simulink model "PRACTICA 1"  (R2024a)
settings: Solver=ode23  StartTime=0.0  StopTime=200  RelTol=1e-3
values from neighbouring files (symbols this model uses):
  g = 9.81    [CONDICIONES.m]
  l1 = 0.3    [CONDICIONES.m]
  l2 = 0.25    [CONDICIONES.m]
  m1 = 0.2    [CONDICIONES.m]
  m2 = 0.1    [CONDICIONES.m]
settings Model: Creator=Charles  LastModifiedBy=JUAN CARLOS
settings SolverCC: AlgebraicLoopSolver=TrustRegion
settings DataIOCC: ReturnWorkspaceOutputs=off
settings DebuggingCC: UnconnectedInputMsg=warning  UnconnectedOutputMsg=warning  UnconnectedLineMsg=warning  ArithmeticOperatorsInVariantConditions=warning
settings ModelReferenceCC: EnableRefExpFcnMdlSchedulingChecks=on
settings SFSimCC: SimUseLocalCustomCode=off  CustomCodeUndefinedFunction=UseInterfaceOnly
settings RTWCC: RTWUseLocalCustomCode=off  GPUComputeCapability=3.5

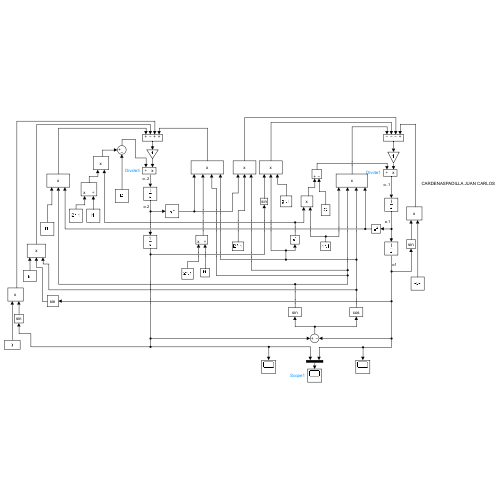
[thumbnail: Simulink's stored preview of the top-level diagram]
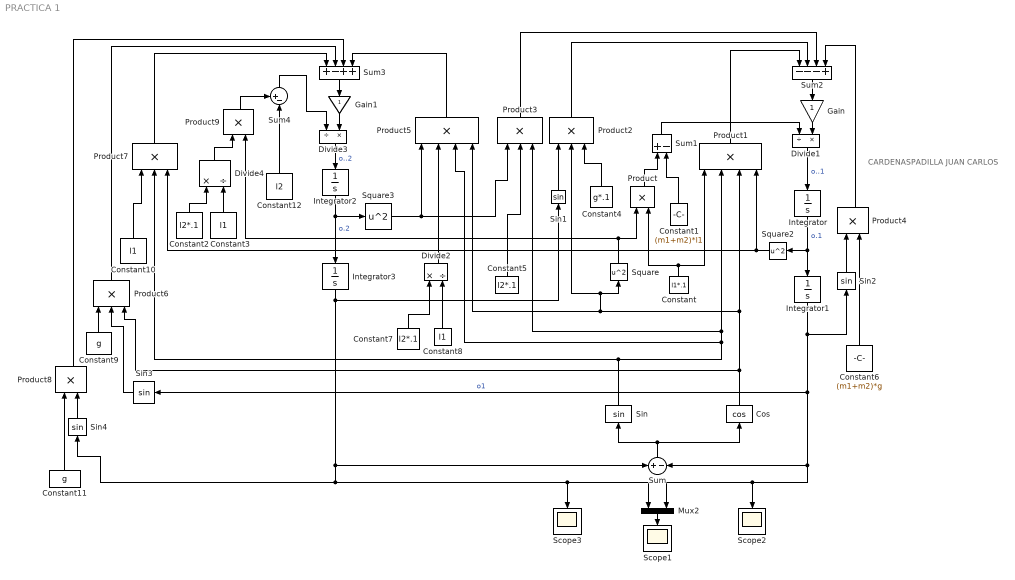
== system PRACTICA 1 ==
  note: CARDENASPADILLA JUAN CARLOS
  Constant : Constant  Value=l1*.1
  Constant1 : Constant  Value=(m1+m2)*l1
  Constant10 : Constant  Value=l1
  Constant11 : Constant  Value=g
  Constant12 : Constant  Value=l2
  Constant2 : Constant  Value=l2*.1
  Constant3 : Constant  Value=l1
  Constant4 : Constant  Value=g*.1
  Constant5 : Constant  Value=l2*.1
  Constant6 : Constant  Value=(m1+m2)*g
  Constant7 : Constant  Value=l2*.1
  Constant8 : Constant  Value=l1
  Constant9 : Constant  Value=g
  Cos : Trigonometry  Operator=cos
  Divide1 : Product  Inputs=/*
  Divide2 : Product  Inputs=*/
  Divide3 : Product  Inputs=/*
  Divide4 : Product  Inputs=*/
  Gain : Gain
  Gain1 : Gain
  Integrator : Integrator
  Integrator1 : Integrator
  Integrator2 : Integrator
  Integrator3 : Integrator  InitialCondition=0.610865
  Mux2 : Mux  Inputs=2
  Product{,4,8..9} (4 alike) : Product
  Product1 : Product  Inputs=4
  Product{2..3,6..7} (4 alike) : Product  Inputs=3
  Product5 : Product  Inputs=4
  Scope1 : Scope
  Scope2 : Scope
  Scope3 : Scope
  Sin{,1..4} (5 alike) : Trigonometry
  Square : Math  Operator=square  SignedPower=on  RndMeth=Zero
  Square2 : Math  Operator=square  SignedPower=on  RndMeth=Zero
  Square3 : Math  Operator=square  SignedPower=on  RndMeth=Zero
  Sum : Sum  Inputs=+-
  Sum1 : Sum  Inputs=+-
  Sum2 : Sum  Inputs=---+
  Sum3 : Sum  Inputs=+-++
  Sum4 : Sum  Inputs=+-|
  wires:
  Gain/1 -> Divide1/2
  Integrator/1 -> Integrator1/1, Square2/1  "o.1"
  Integrator1/1 -> Scope2/1, Mux2/2, Sum/2, Sin3/1, Sin2/1  "o1"
  Integrator2/1 -> Integrator3/1, Square3/1  "o.2"
  Integrator3/1 -> Sin4/1, Mux2/1, Scope3/1, Sum/1, Sin1/1
  Gain1/1 -> Divide3/2
  Sum/1 -> Cos/1, Sin/1
  Cos/1 -> Product6/3, Product2/2, Square/1, Product5/4, Product1/3
  Sin/1 -> Product5/3, Product3/3, Product1/2, Product7/2
  Square/1 -> Product/1, Product9/2
  Constant/1 -> Product1/1, Product/2
  Constant1/1 -> Sum1/2
  Product/1 -> Sum1/1
  Sum1/1 -> Divide1/1
  Divide1/1 -> Integrator/1  "o..1"
  Square2/1 -> Product1/4, Product7/3
  Product1/1 -> Sum2/1
  Sin1/1 -> Product2/1
  Constant4/1 -> Product2/3
  Product2/1 -> Sum2/2
  Constant5/1 -> Product3/2
  Square3/1 -> Product5/1, Product3/1
  Product3/1 -> Sum2/3
  Sin2/1 -> Product4/1
  Constant6/1 -> Product4/2
  Product4/1 -> Sum2/4
  Sum3/1 -> Gain1/1
  Constant8/1 -> Divide2/2
  Constant7/1 -> Divide2/1
  Divide2/1 -> Product5/2
  Product5/1 -> Sum3/4
  Sin3/1 -> Product6/2
  Constant9/1 -> Product6/1
  Constant10/1 -> Product7/1
  Product7/1 -> Sum3/1
  Product6/1 -> Sum3/2
  Sin4/1 -> Product8/2
  Constant11/1 -> Product8/1
  Product8/1 -> Sum3/3
  Divide3/1 -> Integrator2/1  "o..2"
  Constant2/1 -> Divide4/1
  Constant3/1 -> Divide4/2
  Divide4/1 -> Product9/1
  Product9/1 -> Sum4/1
  Constant12/1 -> Sum4/2
  Sum4/1 -> Divide3/1
  Mux2/1 -> Scope1/1
  Sum2/1 -> Gain/1
